simulink model "mrefrobotarm_modified_previous_y_error_previous_u"  (R2018b)
settings: Solver=FixedStepAuto  StartTime=0.0  StopTime=60  RelTol=1e-3  AbsTol=1e-6
undefined symbols (not defined in the file or in its folder): now, sfunxy2, simin
libraries: neural x368, simulink x1
(part 4 of 10)

== system mrefrobotarm_modified_previous_y_error_previous_u/Feed-Forward Neural Network/Layer 2/Delays 1 ==
  "p{2}" : Inport  PortDimensions=64
      mask Display: e = 0.06;c1 = [120 230 180]/255;c2 = ([120 230 180]+0)/(256+128);c3 = ([120 230 180]+128)/(256+128);patch([0 1 1 0],[0 0 1 1],c1);patch([0 1 1 1-e 1-e 0+e],[0 0 1 1-e 0+e 0+e],c2);patch([0 0 1 1-e 0+e 0+e],[0 1 1 1-e 1-e 0+e],c3);plot([0 1 1 0 0],[0 0 1 1 0]);
  mux : Mux  Inputs=1
      mask Display: e = 0.06;c1 = [120 150 230]/255;c2 = ([120 150 230]+0)/383;c3 = ([120 150 230]+128)/383;patch([0 1 1 0],[0 0 1 1],c1);patch([0 1 1 1-e 1-e 0+e],[0 0 1 1-e 0+e 0+e],c2);patch([0 0 1 1-e 0+e 0+e],[0 1 1 1-e 1-e 0+e],c3);plot([0 1 1 0 0],[0 0 1 1 0]);disp('Mux')
  "pd{2,1}" : Outport
      mask Display: e = 0.06;c1 = [120 230 180]/255;c2 = ([120 230 180]+0)/(256+128);c3 = ([120 230 180]+128)/(256+128);patch([0 1 1 0],[0 0 1 1],c1);patch([0 1 1 1-e 1-e 0+e],[0 0 1 1-e 0+e 0+e],c2);patch([0 0 1 1-e 0+e 0+e],[0 1 1 1-e 1-e 0+e],c3);plot([0 1 1 0 0],[0 0 1 1 0]);
  wires:
  "p{2}"/1 -> mux/1
  mux/1 -> "pd{2,1}"/1

== system mrefrobotarm_modified_previous_y_error_previous_u/Feed-Forward Neural Network/Layer 2/LW{2,1} ==
  "ad{2,1}" : Inport  PortDimensions=64
      mask Display: e = 0.06;c1 = [120 230 180]/255;c2 = ([120 230 180]+0)/(256+128);c3 = ([120 230 180]+128)/(256+128);patch([0 1 1 0],[0 0 1 1],c1);patch([0 1 1 1-e 1-e 0+e],[0 0 1 1-e 0+e 0+e],c2);patch([0 0 1 1-e 0+e 0+e],[0 1 1 1-e 1-e 0+e],c3);plot([0 1 1 0 0],[0 0 1 1 0]);
  "IW{2,1}(1,:)'" : Constant  Value=[0.70902502643659703895906432080664671957492828369140625;0.289893825761161572085455873093451373279094696044921875;0.77399117913287185377413379683275707066059112548828125;-0.254483565552355350813940049192751757800579071044921875;-0.2132464167403621824181669808240258134901523590087890625;1.0818376237061553268858915544115006923675537109375;-0.257986054136566222982906992911011911928653717041015625;0.4404195682030509484405911280191503465175628662109375;0.05190454673913254268757810905299265868961811065673828125;-1.365173696978221329345615231432020664215087890625;1.480525983284742164158842570031993091106414794921875;0.58644211967991621836659987820894457399845123291015625;-0.9932291501135288580570659178192727267742156982421875;2.020172164195137565201321194763295352458953857421875;1.6471739763611292772793603944592177867889404296875;0.4224297443399078755277287200442515313625335693359375;0.92210293768368634115262238992727361619472503662109375;-2.948262555483120994637147305184043943881988525390625;-0.80433347580282366084958312058006413280963897705078125;0.567602812764593789296441173064522445201873779296875;0.5868145620206985935141119625768624246120452880859375;-3.609560333111308860765120698488317430019378662109375;0.1508599336051445749529165141211706213653087615966796875;-1.213030270234973340137685227091424167156219482421875;2.461981694343129856150653722579590976238250732421875;1.1618960414544858839036578501691110432147979736328125;1.1077091108865868562816103803925216197967529296875;-1.4366979882742025864672541501931846141815185546875;3.6165728493637772089641657657921314239501953125;0.41538320494401792526417693807161413133144378662109375;3.946229932207245827413544247974641621112823486328125;-1.2393891437019386447815350038581527769565582275390625;-0.4798193754049868697819647422875277698040008544921875;-3.268160362301615773361618266790173947811126708984375;1.1070347513402525319037295048474334180355072021484375;-1.1794116093612301288118260345072485506534576416015625;2.180650521494716276293956980225630104541778564453125;1.8355222794674135311510099199949763715267181396484375;-0.65617861750515416030538062841515056788921356201171875;1.5679112526304119779041457150015048682689666748046875;2.831547341381327242970655788667500019073486328125;1.91789849791212763108205763273872435092926025390625;0.437810642166496510885309589866665191948413848876953125;0.44143457350067816236105500138364732265472412109375;0.04154457606388610446668252507151919417083263397216796875;0.74052180386247290488910266503808088600635528564453125;0.93101034202739796352688017577747814357280731201171875;-1.4433568676521029150450203815125860273838043212890625;-0.306230056170154918415704514700337313115596771240234375;2.440677825397847389155003838823176920413970947265625;0.479909667686399810104802554633351974189281463623046875;1.8956841692554393663527889657416380941867828369140625;0.4919323638232186990393302039592526853084564208984375;-1.184363239840938053504260096815414726734161376953125;-1.0905877987020400343709525259328074753284454345703125;-0.15518967936102245896989870743709616363048553466796875;-2.066133109771171927349087127367965877056121826171875;-0.073856575163838422692919039036496542394161224365234375;-0.91155539025093812455224906443618237972259521484375;0.44930436037192833520492740717600099742412567138671875;-0.321147882217847513430797334876842796802520751953125;-4.58954937701713650000101551995612680912017822265625;-3.135784948035853947345685810432769358158111572265625;-0.81738069857614903401810124705662019550800323486328125]
      mask Display: e = 0.06;c1 = [120 150 230]/255;c2 = ([120 150 230]+0)/383;c3 = ([120 150 230]+128)/383;patch([0 1 1 0],[0 0 1 1],c1);patch([0 1 1 1-e 1-e 0+e],[0 0 1 1-e 0+e 0+e],c2);patch([0 0 1 1-e 0+e 0+e],[0 1 1 1-e 1-e 0+e],c3);plot([0 1 1 0 0],[0 0 1 1 0]);disp('weights');
  Mux : Mux  Inputs=1
      mask Display: e = 0.06;c1 = [120 150 230]/255;c2 = ([120 150 230]+0)/383;c3 = ([120 150 230]+128)/383;patch([0 1 1 0],[0 0 1 1],c1);patch([0 1 1 1-e 1-e 0+e],[0 0 1 1-e 0+e 0+e],c2);patch([0 0 1 1-e 0+e 0+e],[0 1 1 1-e 1-e 0+e],c3);plot([0 1 1 0 0],[0 0 1 1 0]);disp('Mux');
  dotprod1 : neural/Weight Functions/dotprod
  "lz{2,1}" : Outport
      mask Display: e = 0.06;c1 = [120 230 180]/255;c2 = ([120 230 180]+0)/(256+128);c3 = ([120 230 180]+128)/(256+128);patch([0 1 1 0],[0 0 1 1],c1);patch([0 1 1 1-e 1-e 0+e],[0 0 1 1-e 0+e 0+e],c2);patch([0 0 1 1-e 0+e 0+e],[0 1 1 1-e 1-e 0+e],c3);plot([0 1 1 0 0],[0 0 1 1 0]);
  wires:
  "IW{2,1}(1,:)'"/1 -> dotprod1/1
  "ad{2,1}"/1 -> dotprod1/2
  dotprod1/1 -> Mux/1
  Mux/1 -> "lz{2,1}"/1

== system mrefrobotarm_modified_previous_y_error_previous_u/bad/Layer 1/Delays 1 ==
  "p{1}" : Inport  PortDimensions=7
      mask Display: e = 0.06;c1 = [120 230 180]/255;c2 = ([120 230 180]+0)/(256+128);c3 = ([120 230 180]+128)/(256+128);patch([0 1 1 0],[0 0 1 1],c1);patch([0 1 1 1-e 1-e 0+e],[0 0 1 1-e 0+e 0+e],c2);patch([0 0 1 1-e 0+e 0+e],[0 1 1 1-e 1-e 0+e],c3);plot([0 1 1 0 0],[0 0 1 1 0]);
  mux : Mux  Inputs=1
      mask Display: e = 0.06;c1 = [120 150 230]/255;c2 = ([120 150 230]+0)/383;c3 = ([120 150 230]+128)/383;patch([0 1 1 0],[0 0 1 1],c1);patch([0 1 1 1-e 1-e 0+e],[0 0 1 1-e 0+e 0+e],c2);patch([0 0 1 1-e 0+e 0+e],[0 1 1 1-e 1-e 0+e],c3);plot([0 1 1 0 0],[0 0 1 1 0]);disp('Mux')
  "pd{1,1}" : Outport
      mask Display: e = 0.06;c1 = [120 230 180]/255;c2 = ([120 230 180]+0)/(256+128);c3 = ([120 230 180]+128)/(256+128);patch([0 1 1 0],[0 0 1 1],c1);patch([0 1 1 1-e 1-e 0+e],[0 0 1 1-e 0+e 0+e],c2);patch([0 0 1 1-e 0+e 0+e],[0 1 1 1-e 1-e 0+e],c3);plot([0 1 1 0 0],[0 0 1 1 0]);
  wires:
  "p{1}"/1 -> mux/1
  mux/1 -> "pd{1,1}"/1

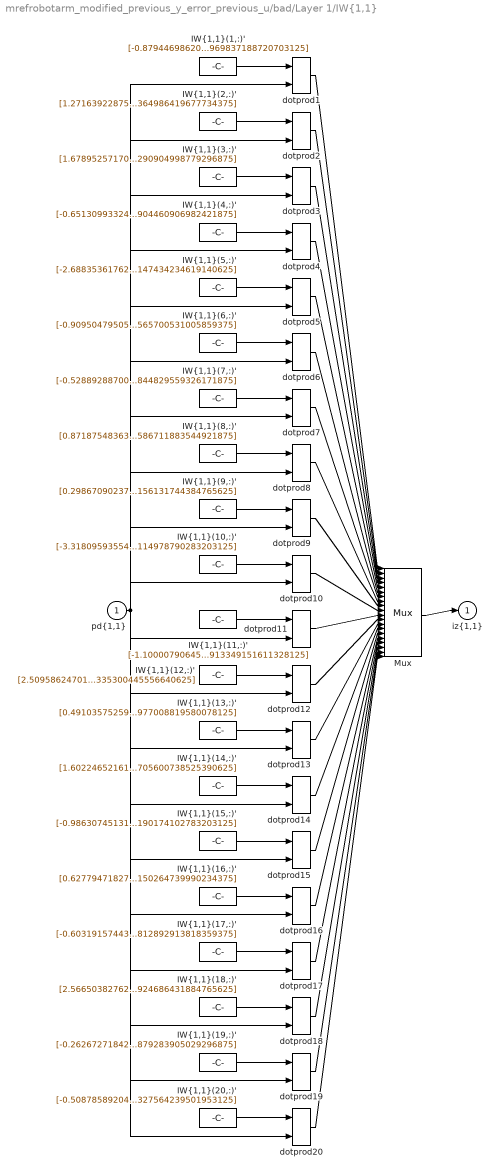
== system mrefrobotarm_modified_previous_y_error_previous_u/bad/Layer 1/IW{1,1} ==
  "pd{1,1}" : Inport  PortDimensions=7
      mask Display: e = 0.06;c1 = [120 230 180]/255;c2 = ([120 230 180]+0)/(256+128);c3 = ([120 230 180]+128)/(256+128);patch([0 1 1 0],[0 0 1 1],c1);patch([0 1 1 1-e 1-e 0+e],[0 0 1 1-e 0+e 0+e],c2);patch([0 0 1 1-e 0+e 0+e],[0 1 1 1-e 1-e 0+e],c3);plot([0 1 1 0 0],[0 0 1 1 0]);
  "IW{1,1}(1,:)'" : Constant  Value=[-0.87944698620385197695981105425744317471981048583984375;0.6913214406650329824088885288801975548267364501953125;0.36853641478774490369829663904965855181217193603515625;1.108092400161881041498190825222991406917572021484375;0.5338655682966078064310977424611337482929229736328125;0.183985876865613795505538519137189723551273345947265625;1.1852539712542775607317935282480902969837188720703125]
      mask Display: e = 0.06;c1 = [120 150 230]/255;c2 = ([120 150 230]+0)/383;c3 = ([120 150 230]+128)/383;patch([0 1 1 0],[0 0 1 1],c1);patch([0 1 1 1-e 1-e 0+e],[0 0 1 1-e 0+e 0+e],c2);patch([0 0 1 1-e 0+e 0+e],[0 1 1 1-e 1-e 0+e],c3);plot([0 1 1 0 0],[0 0 1 1 0]);disp('Weights');
  "IW{1,1}(10,:)'" : Constant  Value=[-3.318095935541440777427624198026023805141448974609375;0.11268487172824741271437432033053482882678508758544921875;-0.0062569322909193890447365760110187693499028682708740234375;-1.1906534479356614131262404043809510767459869384765625;-0.450838125224352903597235808774712495505809783935546875;-0.4867909498363001130627480961265973746776580810546875;-0.473677819968721547372325630931300111114978790283203125]
      mask Display: e = 0.06;c1 = [120 150 230]/255;c2 = ([120 150 230]+0)/383;c3 = ([120 150 230]+128)/383;patch([0 1 1 0],[0 0 1 1],c1);patch([0 1 1 1-e 1-e 0+e],[0 0 1 1-e 0+e 0+e],c2);patch([0 0 1 1-e 0+e 0+e],[0 1 1 1-e 1-e 0+e],c3);plot([0 1 1 0 0],[0 0 1 1 0]);disp('Weights');
  "IW{1,1}(11,:)'" : Constant  Value=[-1.100007906450567674028206965886056423187255859375;-0.76195287073241946274038127739913761615753173828125;0.8481054087517347905844644628814421594142913818359375;1.0723411213635929417620218373485840857028961181640625;-2.070256699841770409165064847911708056926727294921875;-0.97140901063861340158922530463314615190029144287109375;0.7314038794091033413025115805794484913349151611328125]
      mask Display: e = 0.06;c1 = [120 150 230]/255;c2 = ([120 150 230]+0)/383;c3 = ([120 150 230]+128)/383;patch([0 1 1 0],[0 0 1 1],c1);patch([0 1 1 1-e 1-e 0+e],[0 0 1 1-e 0+e 0+e],c2);patch([0 0 1 1-e 0+e 0+e],[0 1 1 1-e 1-e 0+e],c3);plot([0 1 1 0 0],[0 0 1 1 0]);disp('Weights');
  "IW{1,1}(12,:)'" : Constant  Value=[2.509586247011700077536033859360031783580780029296875;-1.115487284079747620779698991100303828716278076171875;-0.14070200355459860919182801808346994221210479736328125;0.891986406405747001002737306407652795314788818359375;0.4999724045135263139627568307332694530487060546875;1.2612737312532191769065548214712180197238922119140625;0.79420503579591328335851585507043637335300445556640625]
      mask Display: e = 0.06;c1 = [120 150 230]/255;c2 = ([120 150 230]+0)/383;c3 = ([120 150 230]+128)/383;patch([0 1 1 0],[0 0 1 1],c1);patch([0 1 1 1-e 1-e 0+e],[0 0 1 1-e 0+e 0+e],c2);patch([0 0 1 1-e 0+e 0+e],[0 1 1 1-e 1-e 0+e],c3);plot([0 1 1 0 0],[0 0 1 1 0]);disp('Weights');
  "IW{1,1}(13,:)'" : Constant  Value=[0.491035752598557417858415874434285797178745269775390625;1.3411235993521495313274272120906971395015716552734375;-0.76492799964221536157538139377720654010772705078125;0.27277669704457718768964014088851399719715118408203125;1.214445003462298444674161146394908428192138671875;0.50441119818881097192075912971631623804569244384765625;0.79296626869284658756242833987926132977008819580078125]
      mask Display: e = 0.06;c1 = [120 150 230]/255;c2 = ([120 150 230]+0)/383;c3 = ([120 150 230]+128)/383;patch([0 1 1 0],[0 0 1 1],c1);patch([0 1 1 1-e 1-e 0+e],[0 0 1 1-e 0+e 0+e],c2);patch([0 0 1 1-e 0+e 0+e],[0 1 1 1-e 1-e 0+e],c3);plot([0 1 1 0 0],[0 0 1 1 0]);disp('Weights');
  "IW{1,1}(14,:)'" : Constant  Value=[1.6022465216123047415663904757821001112461090087890625;0.96990906265602083724530757535831071436405181884765625;0.05233050363256107340159672958179726265370845794677734375;0.9582451471505171181064497432089410722255706787109375;-0.307521778778558907418982926174066960811614990234375;-0.95456583149592810766392858567996881902217864990234375;-1.2941786963526988873951495406799949705600738525390625]
      mask Display: e = 0.06;c1 = [120 150 230]/255;c2 = ([120 150 230]+0)/383;c3 = ([120 150 230]+128)/383;patch([0 1 1 0],[0 0 1 1],c1);patch([0 1 1 1-e 1-e 0+e],[0 0 1 1-e 0+e 0+e],c2);patch([0 0 1 1-e 0+e 0+e],[0 1 1 1-e 1-e 0+e],c3);plot([0 1 1 0 0],[0 0 1 1 0]);disp('Weights');
  "IW{1,1}(15,:)'" : Constant  Value=[-0.986307451317799621648418906261213123798370361328125;1.01896025566066672496390310698188841342926025390625;-0.78087840131964092460492565805907361209392547607421875;-0.4409443105697459230896129156462848186492919921875;-0.611434718287475309494993780390359461307525634765625;-0.342664449270884741149956198569270782172679901123046875;-0.52101083579008655721764853296917863190174102783203125]
      mask Display: e = 0.06;c1 = [120 150 230]/255;c2 = ([120 150 230]+0)/383;c3 = ([120 150 230]+128)/383;patch([0 1 1 0],[0 0 1 1],c1);patch([0 1 1 1-e 1-e 0+e],[0 0 1 1-e 0+e 0+e],c2);patch([0 0 1 1-e 0+e 0+e],[0 1 1 1-e 1-e 0+e],c3);plot([0 1 1 0 0],[0 0 1 1 0]);disp('Weights');
  "IW{1,1}(16,:)'" : Constant  Value=[0.627794718277614460788527139811776578426361083984375;0.29768594171863227426655384988407604396343231201171875;-0.09892951968619574654173476346841198392212390899658203125;-1.4524175729477828422631091598304919898509979248046875;-0.64673503324050518603627324409899301826953887939453125;1.20246938864691710335819152533076703548431396484375;0.09373620823659632728119817102196975611150264739990234375]
      mask Display: e = 0.06;c1 = [120 150 230]/255;c2 = ([120 150 230]+0)/383;c3 = ([120 150 230]+128)/383;patch([0 1 1 0],[0 0 1 1],c1);patch([0 1 1 1-e 1-e 0+e],[0 0 1 1-e 0+e 0+e],c2);patch([0 0 1 1-e 0+e 0+e],[0 1 1 1-e 1-e 0+e],c3);plot([0 1 1 0 0],[0 0 1 1 0]);disp('Weights');
  "IW{1,1}(17,:)'" : Constant  Value=[-0.60319157443413995434156049668672494590282440185546875;0.483580056133551650088264750593225471675395965576171875;-1.1927570300645438106101892117294482886791229248046875;0.346630467947631359937332717890967614948749542236328125;0.63821240914222510109965469382586888968944549560546875;1.381802908054661660486317487084306776523590087890625;-0.38230879298973829971686200224212370812892913818359375]
      mask Display: e = 0.06;c1 = [120 150 230]/255;c2 = ([120 150 230]+0)/383;c3 = ([120 150 230]+128)/383;patch([0 1 1 0],[0 0 1 1],c1);patch([0 1 1 1-e 1-e 0+e],[0 0 1 1-e 0+e 0+e],c2);patch([0 0 1 1-e 0+e 0+e],[0 1 1 1-e 1-e 0+e],c3);plot([0 1 1 0 0],[0 0 1 1 0]);disp('Weights');
  "IW{1,1}(18,:)'" : Constant  Value=[2.566503827622432343247282915399409830570220947265625;-2.4647693855302730270295796799473464488983154296875;-1.1186903830665293479995625602896325290203094482421875;0.332493053566258411901657154885469935834407806396484375;-1.3789757655874208541746384071302600204944610595703125;-0.274444414923749990808943266529240645468235015869140625;-0.01037507375207837034825075761546031571924686431884765625]
      mask Display: e = 0.06;c1 = [120 150 230]/255;c2 = ([120 150 230]+0)/383;c3 = ([120 150 230]+128)/383;patch([0 1 1 0],[0 0 1 1],c1);patch([0 1 1 1-e 1-e 0+e],[0 0 1 1-e 0+e 0+e],c2);patch([0 0 1 1-e 0+e 0+e],[0 1 1 1-e 1-e 0+e],c3);plot([0 1 1 0 0],[0 0 1 1 0]);disp('Weights');
  "IW{1,1}(19,:)'" : Constant  Value=[-0.2626727184248254243215114911436103284358978271484375;0.7055577230445917447099191122106276452541351318359375;0.79050328891379717521914471944910474121570587158203125;0.84480342744452896486251347596407867968082427978515625;0.94305752649468954640354922958067618310451507568359375;0.99337658621110402901166480660322122275829315185546875;-1.396524049770366371348018219578079879283905029296875]
      mask Display: e = 0.06;c1 = [120 150 230]/255;c2 = ([120 150 230]+0)/383;c3 = ([120 150 230]+128)/383;patch([0 1 1 0],[0 0 1 1],c1);patch([0 1 1 1-e 1-e 0+e],[0 0 1 1-e 0+e 0+e],c2);patch([0 0 1 1-e 0+e 0+e],[0 1 1 1-e 1-e 0+e],c3);plot([0 1 1 0 0],[0 0 1 1 0]);disp('Weights');
  "IW{1,1}(2,:)'" : Constant  Value=[1.2716392287569588948059617905528284609317779541015625;-0.9514319304851657221888672211207449436187744140625;-0.84598237599161285604765225798473693430423736572265625;0.126013339313534367125413382382248528301715850830078125;0.92315479318391335805671360503765754401683807373046875;0.36709894804390985623143706106930039823055267333984375;0.7162779711285958139654894694103859364986419677734375]
      mask Display: e = 0.06;c1 = [120 150 230]/255;c2 = ([120 150 230]+0)/383;c3 = ([120 150 230]+128)/383;patch([0 1 1 0],[0 0 1 1],c1);patch([0 1 1 1-e 1-e 0+e],[0 0 1 1-e 0+e 0+e],c2);patch([0 0 1 1-e 0+e 0+e],[0 1 1 1-e 1-e 0+e],c3);plot([0 1 1 0 0],[0 0 1 1 0]);disp('Weights');
  "IW{1,1}(20,:)'" : Constant  Value=[-0.508785892045823029405937631963752210140228271484375;-0.1030420999075026544655742100076167844235897064208984375;1.0756171849409223995053253020159900188446044921875;0.3505326712109260167693491894169710576534271240234375;1.149686115322336998900709659210406243801116943359375;-1.1398513775122964819530579916317947208881378173828125;0.062455236207795923608632193690937128849327564239501953125]
      mask Display: e = 0.06;c1 = [120 150 230]/255;c2 = ([120 150 230]+0)/383;c3 = ([120 150 230]+128)/383;patch([0 1 1 0],[0 0 1 1],c1);patch([0 1 1 1-e 1-e 0+e],[0 0 1 1-e 0+e 0+e],c2);patch([0 0 1 1-e 0+e 0+e],[0 1 1 1-e 1-e 0+e],c3);plot([0 1 1 0 0],[0 0 1 1 0]);disp('Weights');
  "IW{1,1}(3,:)'" : Constant  Value=[1.6789525717025777229451932726078666746616363525390625;0.65473857906108146043067108621471561491489410400390625;-0.60383761111555045442145228662411682307720184326171875;-0.54730088277942334773484844845370389521121978759765625;-0.060930727527578727731327745686940033920109272003173828125;-1.2327148455604823862330476913484744727611541748046875;-0.76349645996291914951115131771075539290904998779296875]
      mask Display: e = 0.06;c1 = [120 150 230]/255;c2 = ([120 150 230]+0)/383;c3 = ([120 150 230]+128)/383;patch([0 1 1 0],[0 0 1 1],c1);patch([0 1 1 1-e 1-e 0+e],[0 0 1 1-e 0+e 0+e],c2);patch([0 0 1 1-e 0+e 0+e],[0 1 1 1-e 1-e 0+e],c3);plot([0 1 1 0 0],[0 0 1 1 0]);disp('Weights');
  "IW{1,1}(4,:)'" : Constant  Value=[-0.6513099332442973121715112938545644283294677734375;1.1299491237335426152554873624467290937900543212890625;0.79824681752819526270315009242040105164051055908203125;0.480407574937419090677082067486480809748172760009765625;-0.61645699309039780899865945684723556041717529296875;-0.351766026995432412594055904264678247272968292236328125;-0.9201863603253961354511147874291054904460906982421875]
      mask Display: e = 0.06;c1 = [120 150 230]/255;c2 = ([120 150 230]+0)/383;c3 = ([120 150 230]+128)/383;patch([0 1 1 0],[0 0 1 1],c1);patch([0 1 1 1-e 1-e 0+e],[0 0 1 1-e 0+e 0+e],c2);patch([0 0 1 1-e 0+e 0+e],[0 1 1 1-e 1-e 0+e],c3);plot([0 1 1 0 0],[0 0 1 1 0]);disp('Weights');
  "IW{1,1}(5,:)'" : Constant  Value=[-2.68835361762342728297880967147648334503173828125;-3.053679159030318945866611102246679365634918212890625;-0.97889991771910767059949876056634820997714996337890625;0.387831467238974825217923125819652341306209564208984375;-1.3858516751735894256825076809036545455455780029296875;-0.97451094154507178490831620365497656166553497314453125;-0.223348099728888416226624258342781104147434234619140625]
      mask Display: e = 0.06;c1 = [120 150 230]/255;c2 = ([120 150 230]+0)/383;c3 = ([120 150 230]+128)/383;patch([0 1 1 0],[0 0 1 1],c1);patch([0 1 1 1-e 1-e 0+e],[0 0 1 1-e 0+e 0+e],c2);patch([0 0 1 1-e 0+e 0+e],[0 1 1 1-e 1-e 0+e],c3);plot([0 1 1 0 0],[0 0 1 1 0]);disp('Weights');
  "IW{1,1}(6,:)'" : Constant  Value=[-0.90950479505752690467801357954158447682857513427734375;1.850358825146404928574384030071087181568145751953125;-0.8322807562609757514593411542591638863086700439453125;-0.52476677260792070622841265503666363656520843505859375;-0.383825988271894680270435173952137120068073272705078125;0.91435479541281294846299942946643568575382232666015625;1.1994728538435237563675173078081570565700531005859375]
      mask Display: e = 0.06;c1 = [120 150 230]/255;c2 = ([120 150 230]+0)/383;c3 = ([120 150 230]+128)/383;patch([0 1 1 0],[0 0 1 1],c1);patch([0 1 1 1-e 1-e 0+e],[0 0 1 1-e 0+e 0+e],c2);patch([0 0 1 1-e 0+e 0+e],[0 1 1 1-e 1-e 0+e],c3);plot([0 1 1 0 0],[0 0 1 1 0]);disp('Weights');
  "IW{1,1}(7,:)'" : Constant  Value=[-0.52889288700968195566787244388251565396785736083984375;-0.27709901066289799320685460770619101822376251220703125;1.032749670097825589465401208144612610340118408203125;-0.74048635978955934522360848859534598886966705322265625;1.0147002932601456581807042311993427574634552001953125;-0.238888444198609495305873906545457430183887481689453125;0.72963317142691053174274884440819732844829559326171875]
      mask Display: e = 0.06;c1 = [120 150 230]/255;c2 = ([120 150 230]+0)/383;c3 = ([120 150 230]+128)/383;patch([0 1 1 0],[0 0 1 1],c1);patch([0 1 1 1-e 1-e 0+e],[0 0 1 1-e 0+e 0+e],c2);patch([0 0 1 1-e 0+e 0+e],[0 1 1 1-e 1-e 0+e],c3);plot([0 1 1 0 0],[0 0 1 1 0]);disp('Weights');
  "IW{1,1}(8,:)'" : Constant  Value=[0.87187548363267330930881371386931277811527252197265625;0.91431308835716718075303788282326422631740570068359375;1.4251563284297201761319229262880980968475341796875;-1.192054376899001066902883394504897296428680419921875;-0.303859440156206972449837167005171068012714385986328125;0.333545341318771948468935306664207018911838531494140625;-0.01144818392031240854300744302918246830813586711883544921875]
      mask Display: e = 0.06;c1 = [120 150 230]/255;c2 = ([120 150 230]+0)/383;c3 = ([120 150 230]+128)/383;patch([0 1 1 0],[0 0 1 1],c1);patch([0 1 1 1-e 1-e 0+e],[0 0 1 1-e 0+e 0+e],c2);patch([0 0 1 1-e 0+e 0+e],[0 1 1 1-e 1-e 0+e],c3);plot([0 1 1 0 0],[0 0 1 1 0]);disp('Weights');
  "IW{1,1}(9,:)'" : Constant  Value=[0.298670902370150981308682958115241490304470062255859375;-1.7941652350290964168522123145521618425846099853515625;-0.7462893223050273139307364544947631657123565673828125;-0.010657999062873950435470504771728883497416973114013671875;-1.51364432339344379130352535867132246494293212890625;0.67930795778262176298767371918074786663055419921875;1.4085468575183048844934319276944734156131744384765625]
      mask Display: e = 0.06;c1 = [120 150 230]/255;c2 = ([120 150 230]+0)/383;c3 = ([120 150 230]+128)/383;patch([0 1 1 0],[0 0 1 1],c1);patch([0 1 1 1-e 1-e 0+e],[0 0 1 1-e 0+e 0+e],c2);patch([0 0 1 1-e 0+e 0+e],[0 1 1 1-e 1-e 0+e],c3);plot([0 1 1 0 0],[0 0 1 1 0]);disp('Weights');
  Mux : Mux  Inputs=20
      mask Display: e = 0.06;c1 = [120 150 230]/255;c2 = ([120 150 230]+0)/383;c3 = ([120 150 230]+128)/383;patch([0 1 1 0],[0 0 1 1],c1);patch([0 1 1 1-e 1-e 0+e],[0 0 1 1-e 0+e 0+e],c2);patch([0 0 1 1-e 0+e 0+e],[0 1 1 1-e 1-e 0+e],c3);plot([0 1 1 0 0],[0 0 1 1 0]);disp('Mux');
  dotprod{1..20} (20 alike) : neural/Weight Functions/dotprod
  "iz{1,1}" : Outport
      mask Display: e = 0.06;c1 = [120 230 180]/255;c2 = ([120 230 180]+0)/(256+128);c3 = ([120 230 180]+128)/(256+128);patch([0 1 1 0],[0 0 1 1],c1);patch([0 1 1 1-e 1-e 0+e],[0 0 1 1-e 0+e 0+e],c2);patch([0 0 1 1-e 0+e 0+e],[0 1 1 1-e 1-e 0+e],c3);plot([0 1 1 0 0],[0 0 1 1 0]);
  wires:
  "IW{1,1}(1,:)'"/1 -> dotprod1/1
  "pd{1,1}"/1 -> dotprod1/2, dotprod2/2, dotprod3/2, dotprod4/2, dotprod5/2, dotprod6/2, dotprod7/2, dotprod8/2, dotprod9/2, dotprod10/2, dotprod11/2, dotprod12/2, dotprod13/2, dotprod14/2, dotprod15/2, dotprod16/2, dotprod17/2, dotprod18/2, dotprod19/2, dotprod20/2
  dotprod1/1 -> Mux/1
  "IW{1,1}(2,:)'"/1 -> dotprod2/1
  dotprod2/1 -> Mux/2
  "IW{1,1}(3,:)'"/1 -> dotprod3/1
  dotprod3/1 -> Mux/3
  "IW{1,1}(4,:)'"/1 -> dotprod4/1
  dotprod4/1 -> Mux/4
  "IW{1,1}(5,:)'"/1 -> dotprod5/1
  dotprod5/1 -> Mux/5
  "IW{1,1}(6,:)'"/1 -> dotprod6/1
  dotprod6/1 -> Mux/6
  "IW{1,1}(7,:)'"/1 -> dotprod7/1
  dotprod7/1 -> Mux/7
  "IW{1,1}(8,:)'"/1 -> dotprod8/1
  dotprod8/1 -> Mux/8
  "IW{1,1}(9,:)'"/1 -> dotprod9/1
  dotprod9/1 -> Mux/9
  "IW{1,1}(10,:)'"/1 -> dotprod10/1
  dotprod10/1 -> Mux/10
  "IW{1,1}(11,:)'"/1 -> dotprod11/1
  dotprod11/1 -> Mux/11
  "IW{1,1}(12,:)'"/1 -> dotprod12/1
  dotprod12/1 -> Mux/12
  "IW{1,1}(13,:)'"/1 -> dotprod13/1
  dotprod13/1 -> Mux/13
  "IW{1,1}(14,:)'"/1 -> dotprod14/1
  dotprod14/1 -> Mux/14
  "IW{1,1}(15,:)'"/1 -> dotprod15/1
  dotprod15/1 -> Mux/15
  "IW{1,1}(16,:)'"/1 -> dotprod16/1
  dotprod16/1 -> Mux/16
  "IW{1,1}(17,:)'"/1 -> dotprod17/1
  dotprod17/1 -> Mux/17
  "IW{1,1}(18,:)'"/1 -> dotprod18/1
  dotprod18/1 -> Mux/18
  "IW{1,1}(19,:)'"/1 -> dotprod19/1
  dotprod19/1 -> Mux/19
  "IW{1,1}(20,:)'"/1 -> dotprod20/1
  dotprod20/1 -> Mux/20
  Mux/1 -> "iz{1,1}"/1

== system mrefrobotarm_modified_previous_y_error_previous_u/bad/Layer 2/Delays 1 ==
  "p{2}" : Inport  PortDimensions=20
      mask Display: e = 0.06;c1 = [120 230 180]/255;c2 = ([120 230 180]+0)/(256+128);c3 = ([120 230 180]+128)/(256+128);patch([0 1 1 0],[0 0 1 1],c1);patch([0 1 1 1-e 1-e 0+e],[0 0 1 1-e 0+e 0+e],c2);patch([0 0 1 1-e 0+e 0+e],[0 1 1 1-e 1-e 0+e],c3);plot([0 1 1 0 0],[0 0 1 1 0]);
  mux : Mux  Inputs=1
      mask Display: e = 0.06;c1 = [120 150 230]/255;c2 = ([120 150 230]+0)/383;c3 = ([120 150 230]+128)/383;patch([0 1 1 0],[0 0 1 1],c1);patch([0 1 1 1-e 1-e 0+e],[0 0 1 1-e 0+e 0+e],c2);patch([0 0 1 1-e 0+e 0+e],[0 1 1 1-e 1-e 0+e],c3);plot([0 1 1 0 0],[0 0 1 1 0]);disp('Mux')
  "pd{2,1}" : Outport
      mask Display: e = 0.06;c1 = [120 230 180]/255;c2 = ([120 230 180]+0)/(256+128);c3 = ([120 230 180]+128)/(256+128);patch([0 1 1 0],[0 0 1 1],c1);patch([0 1 1 1-e 1-e 0+e],[0 0 1 1-e 0+e 0+e],c2);patch([0 0 1 1-e 0+e 0+e],[0 1 1 1-e 1-e 0+e],c3);plot([0 1 1 0 0],[0 0 1 1 0]);
  wires:
  "p{2}"/1 -> mux/1
  mux/1 -> "pd{2,1}"/1
